simulink model "te_test"  (Simulink 2.20)
settings: Solver=ode45  StartTime=0.0  StopTime=2  MaxStep=0.05  RelTol=1e-3
StopFcn:
  | teplot
settings Model: SaveOutput=off  ConsistencyChecking=off  RTWPlaceOutputsASAP=off

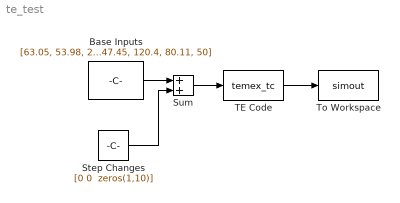
== system te_test ==
  Base Inputs : Constant  Value=[63.05, 53.98, 24.64, 61.31, 22.21, 40.06, 38.10, 46.53, 47.45, 120.4, 80.11, 50]
  Step Changes : Constant  Value="[0 0  zeros(1,10)]"
  Sum : Sum  Inputs=++
  TE Code : S-Function  FunctionName=temex_tc  Parameters=[], [zeros(1,7), 1, zeros(1,12)]  PortCounts=[]  SFunctionModules=''
  To Workspace : ToWorkspace  VariableName=simout  SampleTime=-1
  wires:
  TE Code/1 -> To Workspace/1
  Base Inputs/1 -> Sum/1
  Sum/1 -> TE Code/1
  Step Changes/1 -> Sum/2
